simulink model "Copy_of_DFIG_Dynamic_Model"  (R2013a)
settings: Solver=ode45  StartTime=0.0  StopTime=30  RelTol=1e-3
values from neighbouring files (symbols this model uses):
  B = inv([ ... (first row only)    [WECSConstants.m]
  C = 14e-3    (= 0.014)    [WECSConstants.m]
  f = 60    [WECSConstants.m]
  Ki = 1    [WECSConstants.m]
  Kp = 3    [WECSConstants.m]
  Lg = Xg/wb    (= 0.000189434171015)    [WECSConstants.m]
  Lm = Xm/wb    (= 0.00249597832282)    [WECSConstants.m]
  Lr = Xr/wb    (= 0.00255883889524)    [WECSConstants.m]
  Ls = Xs/wb    (= 0.00255426721724)    [WECSConstants.m]
  P = 6    [WECSConstants.m]
  Pb = (2e6)/3    (= 666666.666667)    [WECSConstants.m]
  sigma = 1-(Lm*Lm)/(Ls*Lr)    (= 0.0468256531123)    [WECSConstants.m]
  Ts = 1    [WECSConstants.m]
  Vb = 690/(3^0.5)    (= 398.371685741)    [WECSConstants.m]
  VDC0 = 1200    [WECSConstants.m]
  wb = 2*pi*f    (= 376.991118431)    [WECSConstants.m]
  ws = wb    (= 376.991118431)    [WECSConstants.m]
  Xm_pu = 3.95279    [WECSConstants.m]
  Xr_pu = Xlr_pu+Xm_pu    (= 4.05234)    [WECSConstants.m]
  Z = [ ... (first row only)    [WECSConstants.m]
  Zb = Vb/Ib    (= 0.23805)    [WECSConstants.m]
undefined symbols (not defined in the file or in its folder): i, Kf, Tcomp
libraries: powerlib_extras x13, powerlib_meascontrol x2, simulink x1
settings Model: Creator=Sony  LastModifiedBy=Sony

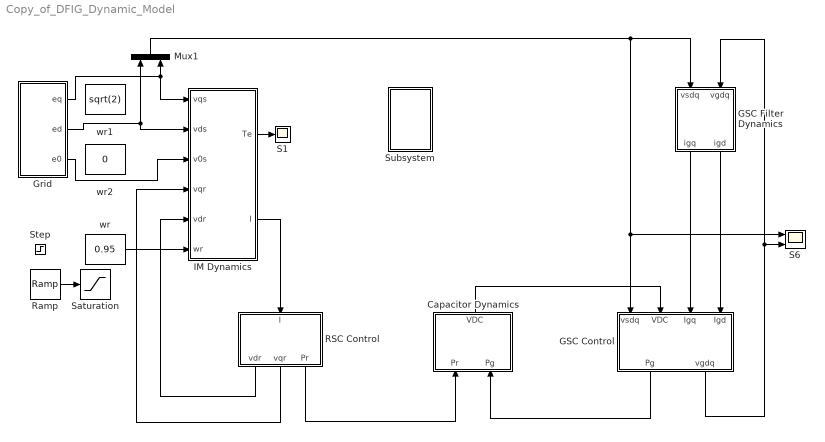
== system Copy_of_DFIG_Dynamic_Model ==
  Capacitor Dynamics : Subsystem
  GSC Control : Subsystem
  GSC Filter Dynamics : Subsystem
  Grid : Subsystem
  IM Dynamics : Subsystem
  Mux1 : Mux  Inputs=2
  RSC Control : Subsystem
  Ramp : simulink/Sources/Ramp  slope=1/5  start=1  X0=0
  S1 : Scope
      settings: SaveName=ScopeData14
  S6 : Scope  NumInputPorts=2
      settings: YMin=0~5.55112e-17  YMax=1.5~1.5  SaveName=ScopeData16
  Saturation : Saturate  UpperLimit=0.95
  Step : Step  Time=0  After=0.95  SampleTime=0
  Subsystem : Subsystem
  wr : Constant  Value=0.95
  wr1 : Constant  Value=sqrt(2)
  wr2 : Constant  Value=0
  wires:
  IM Dynamics/2(I) -> RSC Control/1(I)
  Grid/1(eq) -> IM Dynamics/1(vqs), Mux1/2
  RSC Control/1(vdr) -> IM Dynamics/5(vdr)
  RSC Control/2(vqr) -> IM Dynamics/4(vqr)
  RSC Control/3(Pr) -> Capacitor Dynamics/1(Pr)
  Capacitor Dynamics/1(VDC) -> GSC Control/2(VDC)
  GSC Control/1(Pg) -> Capacitor Dynamics/2(Pg)
  Mux1/1 -> GSC Filter Dynamics/1(vsdq), GSC Control/1(vsdq), S6/1
  GSC Control/2(vgdq) -> GSC Filter Dynamics/2(vgdq), S6/2
  GSC Filter Dynamics/1(igq) -> GSC Control/3(Igq)
  GSC Filter Dynamics/2(igd) -> GSC Control/4(Igd)
  IM Dynamics/1(Te) -> S1/1
  Ramp/1 -> Saturation/1
  wr/1 -> IM Dynamics/6(wr)
  Grid/2(ed) -> IM Dynamics/2(vds), Mux1/1
  Grid/3(e0) -> IM Dynamics/3(v0s)

== system Copy_of_DFIG_Dynamic_Model/Capacitor Dynamics ==
  Pr : Inport
  Pg : Inport  Port=2
  C1 : powerlib_extras/Discrete  Control Blocks/Discrete PI Controller  Kp=0  Ki=1/(C*VDC0)  Par_Limits=[1205 1195]  Init=1200  Ts=50e-6
  G : Gain  Gain=Pb
  G1 : Gain  Gain=1/Vb
  Mux : Mux  Inputs=3
  S2 : Scope
      settings: YMin=1190  YMax=1210  SaveName=ScopeData5
  S3 : Scope
      settings: YMin=-0.5  YMax=0.5  SaveName=ScopeData12
  Sum : Sum  Inputs=|--
  VDC : Outport
  wires:
  Sum/1 -> G/1
  Pr/1 -> Sum/1, Mux/2
  Pg/1 -> Sum/2, Mux/1
  C1/1 -> S2/1, G1/1
  G/1 -> C1/1
  G1/1 -> VDC/1
  [Qg] -> Mux/3
  Mux/1 -> S3/1

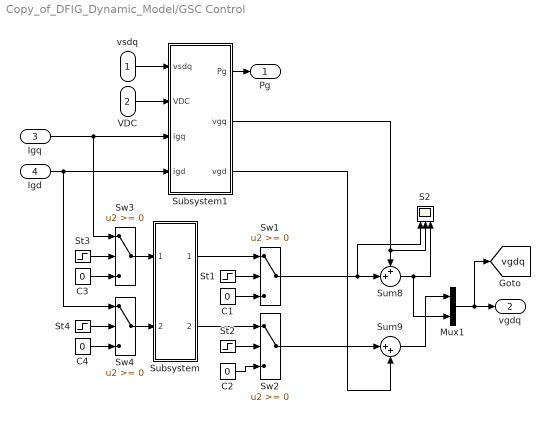
== system Copy_of_DFIG_Dynamic_Model/GSC Control ==
  vsdq : Inport
  VDC : Inport  Port=2
  Igq : Inport  Port=3
  Igd : Inport  Port=4
  C{1..4} (4 alike) : Constant  Value=0
  Mux1 : Mux  Inputs=2
  S2 : Scope  NumInputPorts=3
      settings: YMin=-10~0~1.4137  YMax=10~2~1.4147  SaveName=ScopeData53
  St{1..4} (4 alike) : Step  Time=Tcomp  Before=-1  SampleTime=0
  Subsystem : Subsystem
  Subsystem1 : Subsystem
  Sum8 : Sum  Inputs=++|
  Sum9 : Sum  Inputs=|++
  Sw1 : Switch  SampleTime=Ts
  Sw2 : Switch  SampleTime=Ts
  Sw3 : Switch
  Sw4 : Switch
  Pg : Outport
  vgdq : Outport  Port=2
  tag scope: vgdq=global
  wires:
  Mux1/1 -> [vgdq], vgdq/1
  vsdq/1 -> Subsystem1/1(vsdq)
  VDC/1 -> Subsystem1/2(VDC)
  Subsystem1/1(Pg) -> Pg/1
  Subsystem1/2(vgq) -> S2/2, Sum8/1
  Subsystem1/3(vgd) -> Sum9/2
  St1/1 -> Sw1/2
  C1/1 -> Sw1/3
  Subsystem/1(vgq) -> Sw1/1
  St2/1 -> Sw2/2
  C2/1 -> Sw2/3
  Subsystem/2(vgd) -> Sw2/1
  Sw1/1 -> S2/1, Sum8/2
  Sw2/1 -> Sum9/1
  Sum9/1 -> Mux1/1
  St3/1 -> Sw3/2
  C3/1 -> Sw3/3
  Igq/1 -> Subsystem1/3(igq), Sw3/1
  Sw3/1 -> Subsystem/1(igq)
  St4/1 -> Sw4/2
  C4/1 -> Sw4/3
  Igd/1 -> Sw4/1, Subsystem1/4(igd)
  Sw4/1 -> Subsystem/2(igd)
  Sum8/1 -> S2/3, Mux1/2

== system Copy_of_DFIG_Dynamic_Model/GSC Filter Dynamics ==
  vsdq : Inport
  vgdq : Inport  Port=2
  Add : Sum  Inputs=+-
  Add1 : Sum  Inputs=+-
  Demux : Demux  Outputs=2
  Demux1 : Demux  Outputs=2
  G : Gain
  G1 : Gain  Gain=-Zb/(wb*Lg)
  G2 : Gain  Gain=Zb/(wb*Lg)
  Mux2 : Mux  Inputs=2
  S1 : Scope  NumInputPorts=2
      settings: YMin=1.31236e+20~-5.13413e+16  YMax=1.4505e+20~-4.64517e+16  SaveName=ScopeData31
  S3 : Scope
      settings: YMin=-1  YMax=1  SaveName=ScopeData10
  igq : Outport
  igd : Outport  Port=2
  tag scope: igdq=global
  wires:
  vsdq/1 -> Demux1/1
  vgdq/1 -> Demux/1
  Demux1/2 -> Add/2
  Demux1/1 -> Add1/1
  Mux2/1 -> G/1
  G/1 -> [igdq], S3/1
  Demux/1 -> S1/1, Add1/2
  Demux/2 -> S1/2, Add/1
  G1/1 -> Mux2/2, igd/1
  G2/1 -> Mux2/1, igq/1
  Add/1 -> G1/1
  Add1/1 -> G2/1

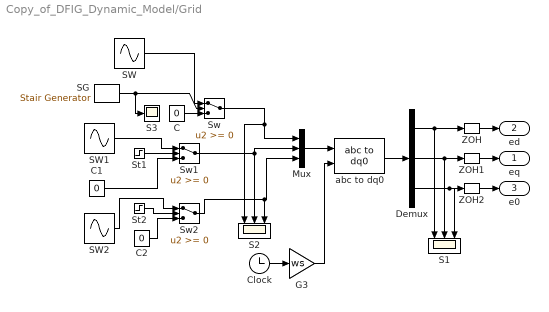
== system Copy_of_DFIG_Dynamic_Model/Grid ==
  C : Constant  Value=0
  C1 : Constant  Value=0
  C2 : Constant  Value=0
  Clock : Clock
  Demux : Demux  Outputs=3
  G3 : Gain  Gain=ws
  Mux : Mux  Inputs=3
  S1 : Scope  NumInputPorts=3
      settings: YMin=-1.5~-1.5~-1.5  YMax=1.5~1.5~1.5  SaveName=ScopeData19
  S2 : Scope  NumInputPorts=3
      settings: YMin=-1.5~-1.5~-1.5  YMax=1.5~1.5~1.5  SaveName=ScopeData21
  S3 : Scope
      settings: YMin=1  YMax=1  SaveName=ScopeData32
  SG : powerlib_meascontrol/Pulse & Signal Generators/Stair Generator  t=[0, 10, 15]  e=[1, -1, 1]  Ts=0
  SW : Sin  Amplitude=sqrt(2)  Frequency=ws  Phase=90*(pi/180)  SampleTime=0
  SW1 : Sin  Amplitude=sqrt(2)  Frequency=ws  Phase=-30*(pi/180)  SampleTime=0
  SW2 : Sin  Amplitude=sqrt(2)  Frequency=ws  Phase=-150*(pi/180)  SampleTime=0
  St1 : Step  Time=0  Before=-1  SampleTime=0
  St2 : Step  Time=0  Before=-1  SampleTime=0
  Sw : Switch
  Sw1 : Switch
  Sw2 : Switch
  ZOH : ZeroOrderHold
  ZOH1 : ZeroOrderHold
  ZOH2 : ZeroOrderHold
  abc to dq0 : powerlib_meascontrol/Transformations/abc to dq0  Alignment=90 degrees behind phase A axis
  eq : Outport
  ed : Outport  Port=2
  e0 : Outport  Port=3
  wires:
  Sw/1 -> S2/1, Mux/1
  Sw1/1 -> Mux/2, S2/2
  Mux/1 -> abc to dq0/1
  Clock/1 -> G3/1
  G3/1 -> abc to dq0/2
  Demux/1 -> ZOH/1, S1/1
  Demux/2 -> S1/2, ZOH1/1
  Demux/3 -> S1/3, ZOH2/1
  abc to dq0/1 -> Demux/1
  Sw2/1 -> S2/3, Mux/3
  SW/1 -> Sw/1
  C/1 -> Sw/3
  St1/1 -> Sw1/2
  C1/1 -> Sw1/3
  SW1/1 -> Sw1/1
  St2/1 -> Sw2/2
  C2/1 -> Sw2/3
  SW2/1 -> Sw2/1
  SG/1 -> S3/1, Sw/2
  ZOH/1 -> ed/1
  ZOH1/1 -> eq/1
  ZOH2/1 -> e0/1

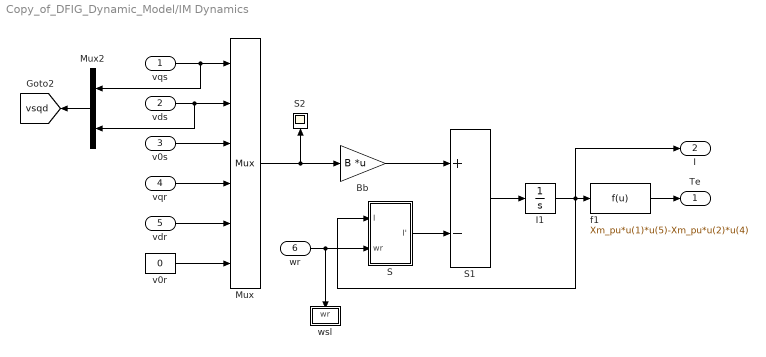
== system Copy_of_DFIG_Dynamic_Model/IM Dynamics ==
  vqs : Inport
  vds : Inport  Port=2
  v0s : Inport  Port=3
  vqr : Inport  Port=4
  vdr : Inport  Port=5
  wr : Inport  Port=6
  Bb : Gain  Gain=B  Multiplication=Matrix(K*u)
  I1 : Integrator  InitialCondition=[-0.5648; 0; 0; 0.578; 0.3585; 0]  UpperSaturationLimit=[2; 2; 2; 2; 2; 2]  LowerSaturationLimit=-[2; 2; 2; 2; 2; 2]
  Mux : Mux  Inputs=6
  Mux2 : Mux  Inputs=2
  S : Subsystem
  S1 : Sum  Inputs=+-
  S2 : Scope
      settings: YMin=950000  YMax=1.05e+06  SaveName=ScopeData8
  f1 : Fcn  Expr=Xm_pu*u(1)*u(5)-Xm_pu*u(2)*u(4)
  v0r : Constant  Value=0
  wsl : Subsystem
  Te : Outport
  I : Outport  Port=2
  tag scope: vsqd=global
  wires:
  S1/1 -> I1/1
  v0s/1 -> Mux/3
  f1/1 -> Te/1
  vdr/1 -> Mux/5
  Mux/1 -> Bb/1, S2/1
  vqr/1 -> Mux/4
  Bb/1 -> S1/1
  S/1(I') -> S1/2
  v0r/1 -> Mux/6
  I1/1 -> I/1, S/1(I), f1/1
  wr/1 -> S/2(wr), wsl/1(wr)
  vqs/1 -> Mux2/1, Mux/1
  vds/1 -> Mux2/2, Mux/2
  Mux2/1 -> [vsqd]

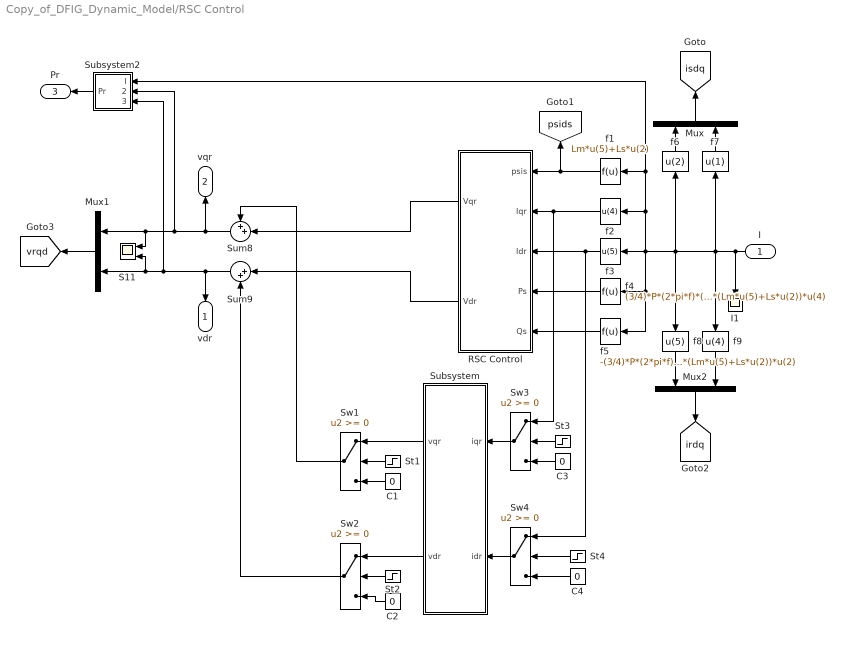
== system Copy_of_DFIG_Dynamic_Model/RSC Control ==
  I : Inport
  C{1..4} (4 alike) : Constant  Value=0
  I1 : Scope
      settings: YMin=-0.6  YMax=0.6
  Mux : Mux  Inputs=2
  Mux1 : Mux  Inputs=2
  Mux2 : Mux  Inputs=2
  RSC Control : Subsystem
  S11 : Scope  NumInputPorts=2
      settings: YMin=-1~-0.01  YMax=1~0.01  SaveName=ScopeData15
  St{1..4} (4 alike) : Step  Time=Tcomp  Before=-1  SampleTime=0
  Subsystem : Subsystem
  Subsystem2 : Subsystem
  Sum8 : Sum  Inputs=++|
  Sum9 : Sum  Inputs=|++
  Sw{1..4} (4 alike) : Switch
  f1 : Fcn  Expr=Lm*u(5)+Ls*u(2)
  f2 : Fcn  Expr=u(4)
  f3 : Fcn  Expr=u(5)
  f4 : Fcn  Expr=(3/4)*P*(2*pi*f)*(Lm/Ls)*(Lm*u(5)+Ls*u(2))*u(4)
  f5 : Fcn  Expr=-(3/4)*P*(2*pi*f)*(Lm*u(5)+Ls*u(2))*u(2)
  f6 : Fcn  Expr=u(2)
  f7 : Fcn  Expr=u(1)
  f8 : Fcn  Expr=u(5)
  f9 : Fcn  Expr=u(4)
  vdr : Outport
  vqr : Outport  Port=2
  Pr : Outport  Port=3
  tag scope: irdq=global, isdq=global, psids=global, vrqd=global
  wires:
  Subsystem2/1(Pr) -> Pr/1
  f1/1 -> RSC Control/1(psis), [psids]
  f4/1 -> RSC Control/4(Ps)
  f5/1 -> RSC Control/5(Qs)
  I/1 -> f5/1, f4/1, Subsystem2/1(I), f1/1, f2/1, f3/1, f8/1, f6/1, f9/1, f7/1, I1/1
  f6/1 -> Mux/1
  f7/1 -> Mux/2
  Mux/1 -> [isdq]
  RSC Control/2(Vdr) -> Sum9/1
  f8/1 -> Mux2/1
  f9/1 -> Mux2/2
  Mux2/1 -> [irdq]
  Subsystem/1(vqr) -> Sw1/1
  Subsystem/2(vdr) -> Sw2/1
  St1/1 -> Sw1/2
  C1/1 -> Sw1/3
  St2/1 -> Sw2/2
  C2/1 -> Sw2/3
  Sw1/1 -> Sum8/1
  Sw2/1 -> Sum9/2
  RSC Control/1(Vqr) -> Sum8/2
  Mux1/1 -> [vrqd]
  Sum8/1 -> Subsystem2/2(vqr), S11/1, Mux1/1, vqr/1
  Sum9/1 -> Subsystem2/3(vdr), S11/2, Mux1/2, vdr/1
  f2/1 -> Sw3/1, RSC Control/2(Iqr)
  St3/1 -> Sw3/2
  C3/1 -> Sw3/3
  Sw3/1 -> Subsystem/1(iqr)
  f3/1 -> Sw4/1, RSC Control/3(Idr)
  St4/1 -> Sw4/2
  C4/1 -> Sw4/3
  Sw4/1 -> Subsystem/2(idr)

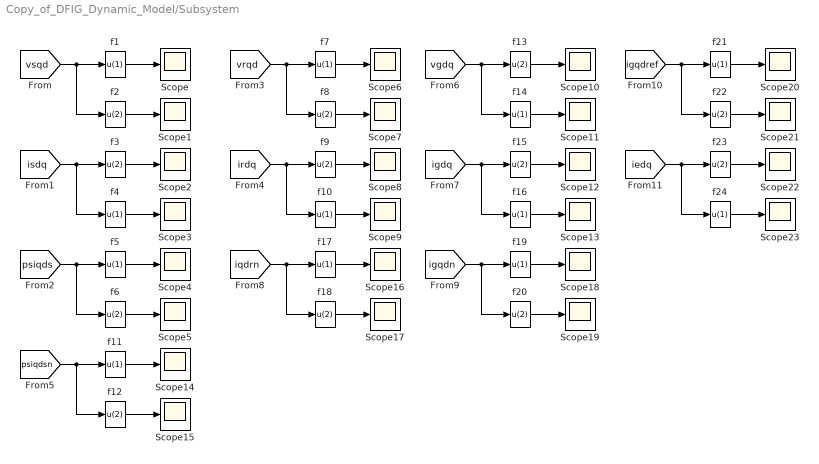
== system Copy_of_DFIG_Dynamic_Model/Subsystem ==
  Scope{,1..23} (24 alike) : Scope
      Scope settings: SaveName=ScopeData23
      Scope1 settings: SaveName=ScopeData26
      Scope10 settings: SaveName=ScopeData40
      Scope11 settings: YMin=0.00902765  YMax=0.00902835  SaveName=ScopeData41
      Scope12 settings: SaveName=ScopeData42
      Scope13 settings: SaveName=ScopeData43
      Scope14 settings: YMin=-0.0015  YMax=0.00125  SaveName=ScopeData38
      Scope15 settings: SaveName=ScopeData39
      Scope16 settings: YMin=-1  YMax=1  SaveName=ScopeData44
      Scope17 settings: YMin=-1  YMax=1  SaveName=ScopeData45
      Scope18 settings: YMin=-1e+25  YMax=1e+25  SaveName=ScopeData46
      Scope19 settings: YMin=-1e+25  YMax=1e+25  SaveName=ScopeData47
      Scope2 settings: SaveName=ScopeData27
      Scope20 settings: YMin=-11.2  YMax=10  SaveName=ScopeData48
      Scope21 settings: YMin=0.00902765  YMax=0.00902835  SaveName=ScopeData49
      Scope22 settings: YMin=-0.6  YMax=-0.275  SaveName=ScopeData50
      Scope23 settings: YMin=-1  YMax=1  SaveName=ScopeData51
      Scope3 settings: SaveName=ScopeData29
      Scope4 settings: SaveName=ScopeData30
      Scope5 settings: YMin=0.0008  YMax=0.001  SaveName=ScopeData33
      Scope6 settings: YMin=0.07000000000000001  YMax=0.08  SaveName=ScopeData34
      Scope7 settings: YMin=-1  YMax=1  SaveName=ScopeData35
      Scope8 settings: SaveName=ScopeData36
      Scope9 settings: SaveName=ScopeData37
  f{1,4..5,7,10..11,14,16..17,19,21,24} (12 alike) : Fcn  Expr=u(1)
  f{2..3,6,8..9,12..13,15,18,20,22..23} (12 alike) : Fcn  Expr=u(2)
  wires:
  [vsqd] -> f2/1, f1/1
  f1/1 -> Scope/1
  f2/1 -> Scope1/1
  [isdq] -> f4/1, f3/1
  f3/1 -> Scope2/1
  f4/1 -> Scope3/1
  [psiqds] -> f6/1, f5/1
  f5/1 -> Scope4/1
  f6/1 -> Scope5/1
  [vrqd] -> f8/1, f7/1
  f7/1 -> Scope6/1
  f8/1 -> Scope7/1
  [irdq] -> f10/1, f9/1
  f9/1 -> Scope8/1
  f10/1 -> Scope9/1
  [vgdq] -> f14/1, f13/1
  f13/1 -> Scope10/1
  f14/1 -> Scope11/1
  [igdq] -> f16/1, f15/1
  f15/1 -> Scope12/1
  f16/1 -> Scope13/1
  [psiqdsn] -> f12/1, f11/1
  f11/1 -> Scope14/1
  f12/1 -> Scope15/1
  [iqdrn] -> f18/1, f17/1
  f17/1 -> Scope16/1
  f18/1 -> Scope17/1
  [igqdn] -> f20/1, f19/1
  f19/1 -> Scope18/1
  f20/1 -> Scope19/1
  [igqdref] -> f22/1, f21/1
  f21/1 -> Scope20/1
  f22/1 -> Scope21/1
  [iedq] -> f24/1, f23/1
  f23/1 -> Scope22/1
  f24/1 -> Scope23/1

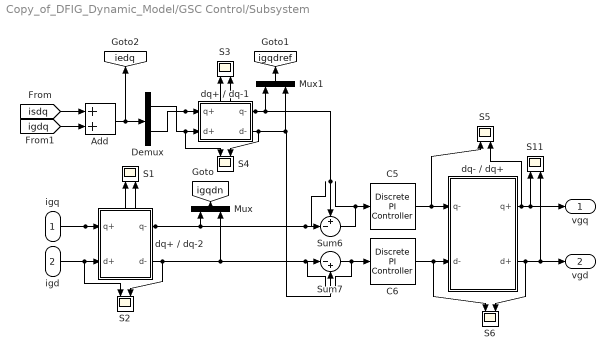
== system Copy_of_DFIG_Dynamic_Model/GSC Control/Subsystem ==
  igq : Inport
  igd : Inport  Port=2
  Add : Sum
  C5 : powerlib_extras/Discrete  Control Blocks/Discrete PI Controller  Kp=Kp  Ki=0  Par_Limits=[10e5 -10e5]  Init=0  Ts=50e-6
  C6 : powerlib_extras/Discrete  Control Blocks/Discrete PI Controller  Kp=Kp  Ki=0  Par_Limits=[10e5 -10e5]  Init=0  Ts=50e-6
  Demux : Demux  Outputs=2
  Mux : Mux  Inputs=2
  Mux1 : Mux  Inputs=2
  S{1..6,11} (7 alike) : Scope  NumInputPorts=2
      S1 settings: YMin=-1~-1  YMax=1~1  SaveName=ScopeData54
      S11 settings: YMin=-1.5~-1.5  YMax=1.5~1.5  SaveName=ScopeData28
      S2 settings: YMin=-1~-1  YMax=1~1  SaveName=ScopeData55
      S3 settings: YMin=-1~-1  YMax=1~1  SaveName=ScopeData56
      S4 settings: YMin=-1~-1  YMax=1~1  SaveName=ScopeData57
      S5 settings: YMin=-1~-1  YMax=1~1  SaveName=ScopeData58
      S6 settings: YMin=-1~-1  YMax=1~1  SaveName=ScopeData59
  Sum6 : Sum  Inputs=+-|
  Sum7 : Sum  Inputs=|-+
  dq+ / dq-1 : Subsystem
  dq+ / dq-2 : Subsystem
  dq- / dq+ : Subsystem
  vgq : Outport
  vgd : Outport  Port=2
  tag scope: iedq=global, igqdn=global, igqdref=global
  wires:
  Demux/1 -> S4/1, dq+ / dq-1/2(d+)
  dq+ / dq-1/2(d-) -> S4/2, Sum7/2, Mux1/2
  [isdq] -> Add/1
  dq- / dq+/1(q+) -> vgq/1, S11/1, S5/2
  dq- / dq+/2(d+) -> S6/2, S11/2, vgd/1
  [igdq] -> Add/2
  dq+ / dq-2/1(q-) -> Sum6/2, Mux/1, S1/2
  Add/1 -> Demux/1, [iedq]
  Sum7/1 -> C6/1
  Sum6/1 -> C5/1
  C5/1 -> S5/1, dq- / dq+/1(q-)
  dq+ / dq-2/2(d-) -> S2/2, Mux/2, Sum7/1
  C6/1 -> S6/1, dq- / dq+/2(d-)
  Demux/2 -> S3/1, dq+ / dq-1/1(q+)
  dq+ / dq-1/1(q-) -> S3/2, Sum6/1, Mux1/1
  igd/1 -> S2/1, dq+ / dq-2/2(d+)
  igq/1 -> S1/1, dq+ / dq-2/1(q+)
  Mux/1 -> [igqdn]
  Mux1/1 -> [igqdref]

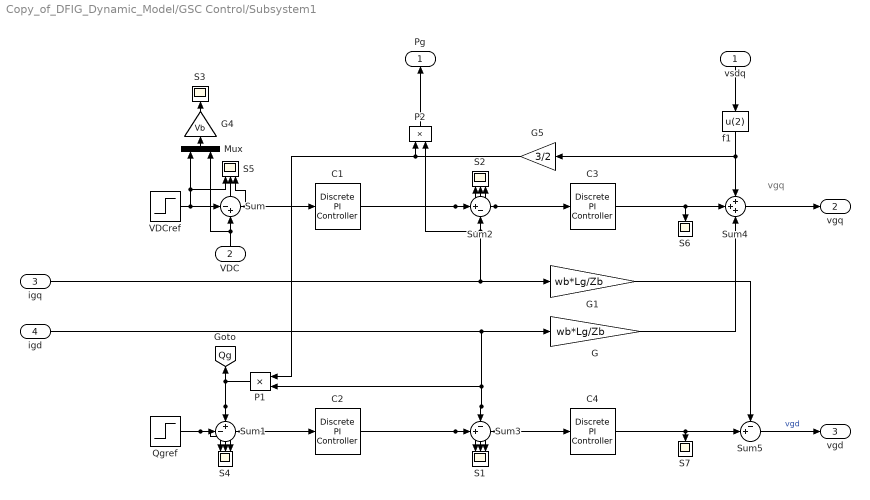
== system Copy_of_DFIG_Dynamic_Model/GSC Control/Subsystem1 ==
  note: vgq
  vsdq : Inport
  VDC : Inport  Port=2
  igq : Inport  Port=3
  igd : Inport  Port=4
  C1 : powerlib_extras/Discrete  Control Blocks/Discrete PI Controller  Kp=Kp  Ki=Ki  Par_Limits=[10e5 -10e5]  Init=0  Ts=Ts
  C2 : powerlib_extras/Discrete  Control Blocks/Discrete PI Controller  Kp=Kp  Ki=Ki  Par_Limits=[10e5 -10e5]  Init=0  Ts=Ts
  C3 : powerlib_extras/Discrete  Control Blocks/Discrete PI Controller  Kp=Kp  Ki=Ki  Par_Limits=[1e6 -1e6]  Init=0  Ts=Ts
  C4 : powerlib_extras/Discrete  Control Blocks/Discrete PI Controller  Kp=Kp  Ki=Ki  Par_Limits=[1e6 -1e6]  Init=0  Ts=Ts
  G : Gain  Gain=wb*Lg/Zb
  G1 : Gain  Gain=wb*Lg/Zb
  G4 : Gain  Gain=Vb
  G5 : Gain  Gain=3/2
  Mux : Mux  Inputs=2
  P1 : Product
  P2 : Product
  Qgref : Step  Time=0  After=0  SampleTime=0
  S{1..2,4..5} (4 alike) : Scope  NumInputPorts=3
      S1 settings: YMin=-1.05e+06~-4.11888e+22~3.7266e+22  YMax=-950000~-3.7266e+22~4.11888e+22  SaveName=ScopeData6
      S2 settings: YMin=0.0357706~-5.87597e+28~5.31635e+28  YMax=0.039536~-5.31635e+28~5.87597e+28  SaveName=ScopeData2
      S4 settings: YMin=-0.25~-0.25~-0.25  YMax=0.25~0.25~0.25  SaveName=ScopeData9
      S5 settings: YMin=2.99~2.99~-0.02  YMax=3.04~3.04~0.02  SaveName=ScopeData11
  S3 : Scope
      settings: YMin=1190  YMax=1210  SaveName=ScopeData22
  S6 : Scope
      settings: TimeRange=0.1  YMin=-1  YMax=1  SaveName=ScopeData24
  S7 : Scope
      settings: TimeRange=50  YMin=-1  YMax=1  SaveName=ScopeData25
  Sum : Sum  Inputs=|-+
  Sum1 : Sum  Inputs=+-|
  Sum2 : Sum  Inputs=|+-
  Sum3 : Sum  Inputs=-+|
  Sum4 : Sum  Inputs=+++
  Sum5 : Sum  Inputs=-+|
  VDCref : Step  Time=0  Before=1200/Vb  After=1200/Vb  SampleTime=0
  f1 : Fcn  Expr=u(2)
  Pg : Outport
  vgq : Outport  Port=2
  vgd : Outport  Port=3
  tag scope: Qg=global
  wires:
  P1/1 -> S4/2, Sum1/1, [Qg]
  Sum3/1 -> C4/1, S1/3
  Sum2/1 -> C3/1, S2/3
  C2/1 -> S1/1, Sum3/2
  VDCref/1 -> S5/1, Mux/1, Sum/1
  VDC/1 -> Mux/2, S5/2, Sum/2
  G5/1 -> P1/1, P2/1
  Sum1/1 -> C2/1, S4/3
  C1/1 -> Sum2/1, S2/1
  C4/1 -> Sum5/2, S7/1
  Qgref/1 -> S4/1, Sum1/2
  G4/1 -> S3/1
  C3/1 -> S6/1, Sum4/2
  G1/1 -> Sum5/1
  vsdq/1 -> f1/1
  Sum5/1 -> vgd/1  "vgd"
  G/1 -> Sum4/3
  Mux/1 -> G4/1
  Sum/1 -> C1/1, S5/3
  f1/1 -> Sum4/1, G5/1
  P2/1 -> Pg/1
  Sum4/1 -> vgq/1
  igq/1 -> S2/2, P2/2, Sum2/2, G1/1
  igd/1 -> Sum3/1, S1/2, P1/2, G/1

== system Copy_of_DFIG_Dynamic_Model/IM Dynamics/S ==
  I : Inport
  wr : Inport  Port=2
  G1 : Gain  Gain=Z  Multiplication=Matrix(K*u)
  G2 : Gain  Gain=B  Multiplication=Matrix(K*u)
  G3 : Gain  Gain=[0 0 0 0 0 0;0 0 0 0 0 0;0 0 0 0 0 0;0 -Xm_pu 0 0 -Xr_pu 0;Xm_pu 0 0 Xr_pu 0 0;0 0 0 0 0 0]
  Matrix Sum : Sum
  P : Product  Multiplication=Matrix(*)
  I' : Outport
  wires:
  G2/1 -> I'/1
  P/1 -> Matrix Sum/2
  Matrix Sum/1 -> G2/1
  G3/1 -> P/1
  G1/1 -> Matrix Sum/1
  I/1 -> P/2, G1/1
  wr/1 -> G3/1

== system Copy_of_DFIG_Dynamic_Model/IM Dynamics/wsl ==
  wr : Inport
  Add1 : Sum  Inputs=+-
  Gain : Gain  Gain=1/wb
  Scope1 : Scope
      settings: YMin=0.9025  YMax=0.9975  SaveName=ScopeData13
  Scope2 : Scope
      settings: YMin=0.0475  YMax=0.0525  SaveName=ScopeData18
  wr1 : Constant
  tag scope: wsl=global
  wires:
  wr/1 -> Scope1/1, Add1/2
  Add1/1 -> Scope2/1, [wsl]
  [we] -> Gain/1
  wr1/1 -> Add1/1

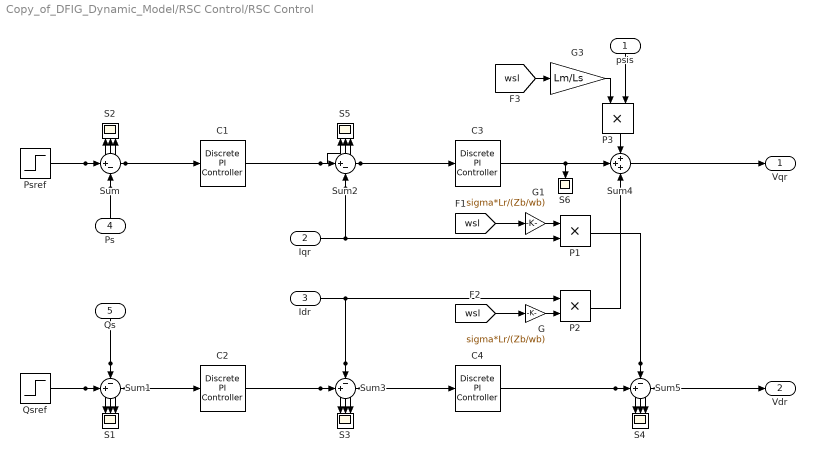
== system Copy_of_DFIG_Dynamic_Model/RSC Control/RSC Control ==
  psis : Inport
  Iqr : Inport  Port=2
  Idr : Inport  Port=3
  Ps : Inport  Port=4
  Qs : Inport  Port=5
  C1 : powerlib_extras/Discrete  Control Blocks/Discrete PI Controller  Kp=Kp  Ki=Ki  Par_Limits=[10e5 -10e5]  Init=0  Ts=50e-6
  C2 : powerlib_extras/Discrete  Control Blocks/Discrete PI Controller  Kp=Kp  Ki=Ki  Par_Limits=[10e5 -10e5]  Init=0  Ts=50e-6
  C3 : powerlib_extras/Discrete  Control Blocks/Discrete PI Controller  Kp=Kp  Ki=Ki  Par_Limits=[10e5 -10e5]  Init=0.0724  Ts=50e-6
  C4 : powerlib_extras/Discrete  Control Blocks/Discrete PI Controller  Kp=Kp  Ki=Ki  Par_Limits=[10e5 -10e5]  Init=1.968e-3  Ts=50e-6
  G : Gain  Gain=sigma*Lr/(Zb/wb)
  G1 : Gain  Gain=sigma*Lr/(Zb/wb)
  G3 : Gain  Gain=Lm/Ls
  P1 : Product
  P2 : Product
  P3 : Product
  Psref : Step  Time=0  Before=0.95*0.95*0.95  After=0.95*0.95*0.95  SampleTime=0
  Qsref : Step  Time=0  After=0  SampleTime=0
  S{1..5} (5 alike) : Scope  NumInputPorts=3
      S1 settings: YMin=-1~-1~-1  YMax=1~1~1  SaveName=ScopeData4
      S2 settings: YMin=0.814506~0.6~-0.3  YMax=0.900244~1.15~0.25  SaveName=ScopeData3
      S3 settings: YMin=0.358236~0.358234~7.5e-07  YMax=0.358241~0.358239~3e-06  SaveName=ScopeData7
      S4 settings: YMin=0.00196795~0.00548418~-0.00351623  YMax=0.00196805~0.00548419~-0.00351613  SaveName=ScopeData17
      S5 settings: YMin=0.5772~0.5776~-0.0005  YMax=0.5789~0.57845~0.0005  SaveName=ScopeData20
  S6 : Scope
      settings: YMin=0.0723587  YMax=0.0723622
  Sum : Sum  Inputs=|+-
  Sum1 : Sum  Inputs=-+|
  Sum2 : Sum  Inputs=|+-
  Sum3 : Sum  Inputs=-+|
  Sum4 : Sum  Inputs=+++
  Sum5 : Sum  Inputs=-+|
  Vqr : Outport
  Vdr : Outport  Port=2
  wires:
  Psref/1 -> S2/1, Sum/1
  Ps/1 -> S2/2, Sum/2
  Qsref/1 -> S1/1, Sum1/2
  Qs/1 -> S1/2, Sum1/1
  Sum/1 -> C1/1, S2/3
  P3/1 -> Sum4/1
  Sum3/1 -> C4/1, S3/3
  G1/1 -> P1/1
  Sum2/1 -> C3/1, S5/3
  Sum1/1 -> C2/1, S1/3
  C4/1 -> S4/1, Sum5/2
  Iqr/1 -> S5/2, Sum2/2, P1/2
  Idr/1 -> S3/2, Sum3/1, P2/1
  C2/1 -> S3/1, Sum3/2
  C3/1 -> S6/1, Sum4/2
  Sum4/1 -> Vqr/1
  Sum5/1 -> Vdr/1, S4/3
  [wsl] -> G1/1
  [wsl] -> G/1
  P1/1 -> S4/2, Sum5/1
  P2/1 -> Sum4/3
  G3/1 -> P3/1
  psis/1 -> P3/2
  [wsl] -> G3/1
  C1/1 -> S5/1, Sum2/1
  G/1 -> P2/2

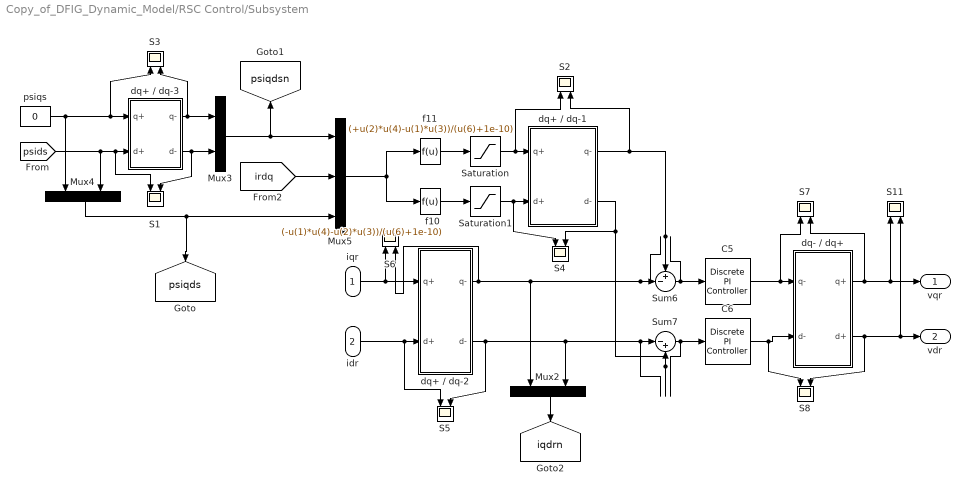
== system Copy_of_DFIG_Dynamic_Model/RSC Control/Subsystem ==
  iqr : Inport
  idr : Inport  Port=2
  C5 : powerlib_extras/Discrete  Control Blocks/Discrete PI Controller  Kp=Kp  Ki=Ki  Par_Limits=[10e5 -10e5]  Init=0  Ts=50e-6
  C6 : powerlib_extras/Discrete  Control Blocks/Discrete PI Controller  Kp=Kp  Ki=Ki  Par_Limits=[10e5 -10e5]  Init=0  Ts=50e-6
  Mux2 : Mux  Inputs=2
  Mux3 : Mux  Inputs=2
  Mux4 : Mux  Inputs=2
  Mux5 : Mux  Inputs=3
  S{1..8,11} (9 alike) : Scope  NumInputPorts=2
      S1 settings: YMin=-1~-1  YMax=1~1  SaveName=ScopeData61
      S11 settings: YMin=-0.5~-0.5  YMax=1.5~1.5  SaveName=ScopeData28
      S2 settings: YMin=-1~-1  YMax=1~1  SaveName=ScopeData62
      S3 settings: YMin=-1~-1  YMax=1~1  SaveName=ScopeData60
      S4 settings: YMin=-1~-1  YMax=1~1  SaveName=ScopeData63
      S5 settings: YMin=-1~-0.0009  YMax=1~0.0011  SaveName=ScopeData64
      S6 settings: YMin=-1~-1  YMax=1~1  SaveName=ScopeData65
      S7 settings: YMin=-1~-1  YMax=1~1  SaveName=ScopeData66
      S8 settings: YMin=-1~-1  YMax=1~1  SaveName=ScopeData67
  Saturation : Saturate  UpperLimit=1e6  LowerLimit=-1e6
  Saturation1 : Saturate  UpperLimit=1e6  LowerLimit=-1e6
  Sum6 : Sum  Inputs=+-|
  Sum7 : Sum  Inputs=|-+
  dq+ / dq-1 : Subsystem
  dq+ / dq-2 : Subsystem
  dq+ / dq-3 : Subsystem
  dq- / dq+ : Subsystem
  f10 : Fcn  Expr=(-u(1)*u(4)-u(2)*u(3))/(u(6)+1e-10)
  f11 : Fcn  Expr=(+u(2)*u(4)-u(1)*u(3))/(u(6)+1e-10)
  psiqs : Constant  Value=0
  vqr : Outport
  vdr : Outport  Port=2
  tag scope: iqdrn=global, psiqds=global, psiqdsn=global
  wires:
  dq+ / dq-1/2(d-) -> S4/2, Sum7/2
  dq- / dq+/1(q+) -> S7/2, vqr/1, S11/1
  dq- / dq+/2(d+) -> S8/2, vdr/1, S11/2
  dq+ / dq-2/1(q-) -> Sum6/2, Mux2/1, S6/2
  Sum7/1 -> C6/1
  Sum6/1 -> C5/1
  C5/1 -> S7/1, dq- / dq+/1(q-)
  dq+ / dq-2/2(d-) -> S5/2, Sum7/1, Mux2/2
  C6/1 -> S8/1, dq- / dq+/2(d-)
  dq+ / dq-1/1(q-) -> S2/2, Sum6/1
  idr/1 -> S5/1, dq+ / dq-2/2(d+)
  psiqs/1 -> S3/1, dq+ / dq-3/1(q+), Mux4/1
  [psids] -> S1/1, dq+ / dq-3/2(d+), Mux4/2
  dq+ / dq-3/1(q-) -> S3/2, Mux3/1
  dq+ / dq-3/2(d-) -> S1/2, Mux3/2
  Mux3/1 -> [psiqdsn], Mux5/1
  [irdq] -> Mux5/2
  Mux5/1 -> f11/1, f10/1
  Mux4/1 -> [psiqds], Mux5/3
  f11/1 -> Saturation/1
  f10/1 -> Saturation1/1
  Mux2/1 -> [iqdrn]
  Saturation/1 -> S2/1, dq+ / dq-1/1(q+)
  Saturation1/1 -> S4/1, dq+ / dq-1/2(d+)
  iqr/1 -> S6/1, dq+ / dq-2/1(q+)

== system Copy_of_DFIG_Dynamic_Model/RSC Control/Subsystem2 ==
  I : Inport
  vqr : Inport  Port=2
  vdr : Inport  Port=3
  A : Sum
  G : Gain  Gain=3/2
  P1 : Product
  P2 : Product
  f6 : Fcn  Expr=u(4)
  f7 : Fcn  Expr=u(5)
  Pr : Outport
  wires:
  P2/1 -> A/2
  G/1 -> Pr/1
  f6/1 -> P1/1
  I/1 -> f7/1, f6/1
  P1/1 -> A/1
  f7/1 -> P2/1
  vdr/1 -> P2/2
  vqr/1 -> P1/2
  A/1 -> G/1

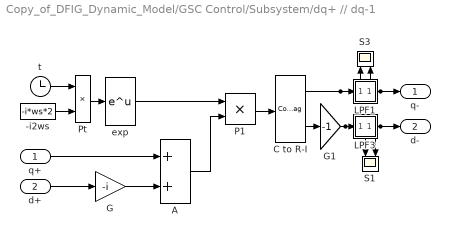
== system Copy_of_DFIG_Dynamic_Model/GSC Control/Subsystem/dq+ // dq-1 ==
  q+ : Inport
  d+ : Inport  Port=2
  -i2ws : Constant  Value=-i*ws*2
  A : Sum
  C to R-I : ComplexToRealImag
  G : Gain  Gain=-i
  G1 : Gain  Gain=-1
  LPF1 : Subsystem
  LPF3 : Subsystem
  P1 : Product
  Pt : Product
  S1 : Scope  NumInputPorts=2
      settings: YMin=-1~-1  YMax=1~1  SaveName=ScopeData69
  S3 : Scope  NumInputPorts=2
      settings: YMin=-1~-1  YMax=1~1  SaveName=ScopeData68
  exp : Math  OutputSignalType=complex  SaturateOnIntegerOverflow=on
  t : Clock
  q- : Outport
  d- : Outport  Port=2
  wires:
  C to R-I/2 -> G1/1
  t/1 -> Pt/1
  -i2ws/1 -> Pt/2
  Pt/1 -> exp/1
  exp/1 -> P1/1
  G/1 -> A/2
  q+/1 -> A/1
  A/1 -> P1/2
  P1/1 -> C to R-I/1
  d+/1 -> G/1
  C to R-I/1 -> LPF1/1(I), S3/1
  G1/1 -> LPF3/1(I), S1/1
  LPF1/1(O) -> q-/1, S3/2
  LPF3/1(O) -> d-/1, S1/2

== system Copy_of_DFIG_Dynamic_Model/GSC Control/Subsystem/dq+ // dq-2 ==
  q+ : Inport
  d+ : Inport  Port=2
  -i2ws : Constant  Value=-i*ws*2
  A : Sum
  C to R-I : ComplexToRealImag
  G : Gain  Gain=-i
  G1 : Gain  Gain=-1
  LPF1 : Subsystem
  LPF3 : Subsystem
  P1 : Product
  Pt : Product
  S11 : Scope  NumInputPorts=2
      settings: YMin=-0.1~-0.01  YMax=0.1~0.01  SaveName=ScopeData52
  S3 : Scope  NumInputPorts=2
      settings: YMin=-1~-0.01  YMax=1~0.01  SaveName=ScopeData70
  exp : Math  OutputSignalType=complex  SaturateOnIntegerOverflow=on
  t : Clock
  q- : Outport
  d- : Outport  Port=2
  wires:
  C to R-I/2 -> G1/1
  t/1 -> Pt/1
  -i2ws/1 -> Pt/2
  Pt/1 -> exp/1
  exp/1 -> P1/1
  G/1 -> A/2
  q+/1 -> A/1
  A/1 -> P1/2
  P1/1 -> C to R-I/1
  d+/1 -> G/1
  C to R-I/1 -> LPF1/1(I), S11/1
  G1/1 -> LPF3/1(I), S3/1
  LPF1/1(O) -> S11/2, q-/1
  LPF3/1(O) -> d-/1, S3/2

== system Copy_of_DFIG_Dynamic_Model/GSC Control/Subsystem/dq- // dq+ ==
  q- : Inport
  d- : Inport  Port=2
  Add : Sum
  Complex to Real-Imag : ComplexToRealImag
  Gain : Gain  Gain=-i
  Gain1 : Gain  Gain=-1
  LPF2 : Subsystem
  LPF4 : Subsystem
  Product : Product
  Product1 : Product
  S1 : Scope  NumInputPorts=2
      settings: YMin=-1~-1  YMax=1~1  SaveName=ScopeData72
  S3 : Scope  NumInputPorts=2
      settings: YMin=-1~-1  YMax=1~1  SaveName=ScopeData71
  exp : Math  SaturateOnIntegerOverflow=on
  i2ws : Constant  Value=i*ws*2
  t : Clock
  q+ : Outport
  d+ : Outport  Port=2
  wires:
  Complex to Real-Imag/2 -> Gain1/1
  t/1 -> Product/1
  i2ws/1 -> Product/2
  Product/1 -> exp/1
  exp/1 -> Product1/1
  d-/1 -> Gain/1
  Gain/1 -> Add/2
  q-/1 -> Add/1
  Add/1 -> Product1/2
  Product1/1 -> Complex to Real-Imag/1
  Complex to Real-Imag/1 -> LPF4/1(I), S3/1
  Gain1/1 -> LPF2/1(I), S1/1
  LPF4/1(O) -> S3/2, q+/1
  LPF2/1(O) -> S1/2, d+/1

== system Copy_of_DFIG_Dynamic_Model/RSC Control/Subsystem/dq+ // dq-1 ==
  q+ : Inport
  d+ : Inport  Port=2
  -i2ws : Constant  Value=-i*ws*2
  A : Sum
  C to R-I : ComplexToRealImag
  G : Gain  Gain=-i
  G1 : Gain  Gain=-1
  LPF1 : Subsystem
  LPF3 : Subsystem
  P1 : Product
  Pt : Product
  S1 : Scope  NumInputPorts=2
      settings: YMin=-1~-1  YMax=1~1  SaveName=ScopeData74
  S3 : Scope  NumInputPorts=2
      settings: YMin=-1~-1  YMax=1~1  SaveName=ScopeData73
  exp : Math  OutputSignalType=complex  SaturateOnIntegerOverflow=on
  t : Clock
  q- : Outport
  d- : Outport  Port=2
  wires:
  C to R-I/2 -> G1/1
  t/1 -> Pt/1
  -i2ws/1 -> Pt/2
  Pt/1 -> exp/1
  exp/1 -> P1/1
  G/1 -> A/2
  q+/1 -> A/1
  A/1 -> P1/2
  P1/1 -> C to R-I/1
  d+/1 -> G/1
  C to R-I/1 -> LPF1/1(I), S3/1
  G1/1 -> LPF3/1(I), S1/1
  LPF1/1(O) -> q-/1, S3/2
  LPF3/1(O) -> d-/1, S1/2

== system Copy_of_DFIG_Dynamic_Model/RSC Control/Subsystem/dq+ // dq-2 ==
  q+ : Inport
  d+ : Inport  Port=2
  -i2ws : Constant  Value=-i*ws*2
  A : Sum
  C to R-I : ComplexToRealImag
  G : Gain  Gain=-i
  G1 : Gain  Gain=-1
  LPF1 : Subsystem
  LPF3 : Subsystem
  P1 : Product
  Pt : Product
  S1 : Scope  NumInputPorts=2
      settings: YMin=-1~-1  YMax=1~1  SaveName=ScopeData76
  S3 : Scope  NumInputPorts=2
      settings: YMin=-1~-1  YMax=1~1  SaveName=ScopeData75
  exp : Math  OutputSignalType=complex  SaturateOnIntegerOverflow=on
  t : Clock
  q- : Outport
  d- : Outport  Port=2
  wires:
  C to R-I/2 -> G1/1
  t/1 -> Pt/1
  -i2ws/1 -> Pt/2
  Pt/1 -> exp/1
  exp/1 -> P1/1
  G/1 -> A/2
  q+/1 -> A/1
  A/1 -> P1/2
  P1/1 -> C to R-I/1
  d+/1 -> G/1
  C to R-I/1 -> LPF1/1(I), S3/1
  G1/1 -> LPF3/1(I), S1/1
  LPF1/1(O) -> S3/2, q-/1
  LPF3/1(O) -> S1/2, d-/1

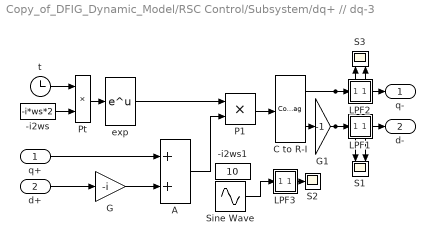
== system Copy_of_DFIG_Dynamic_Model/RSC Control/Subsystem/dq+ // dq-3 ==
  q+ : Inport
  d+ : Inport  Port=2
  -i2ws : Constant  Value=-i*ws*2
  -i2ws1 : Constant  Value=10
  A : Sum
  C to R-I : ComplexToRealImag
  G : Gain  Gain=-i
  G1 : Gain  Gain=-1
  LPF1 : Subsystem
  LPF2 : Subsystem
  LPF3 : Subsystem
  P1 : Product
  Pt : Product
  S1 : Scope  NumInputPorts=2
      settings: YMin=-1~-1  YMax=1~1  SaveName=ScopeData78
  S2 : Scope
      settings: YMin=-4  YMax=6  SaveName=ScopeData81
  S3 : Scope  NumInputPorts=2
      settings: YMin=-1~-1  YMax=1~1  SaveName=ScopeData77
  Sine Wave : Sin  Amplitude=10  Bias=1  Frequency=2*pi*30  SampleTime=0
  exp : Math  OutputSignalType=complex  SaturateOnIntegerOverflow=on
  t : Clock
  q- : Outport
  d- : Outport  Port=2
  wires:
  C to R-I/2 -> G1/1
  t/1 -> Pt/1
  -i2ws/1 -> Pt/2
  Pt/1 -> exp/1
  exp/1 -> P1/1
  G/1 -> A/2
  q+/1 -> A/1
  A/1 -> P1/2
  P1/1 -> C to R-I/1
  d+/1 -> G/1
  C to R-I/1 -> LPF2/1(I), S3/1
  G1/1 -> LPF1/1(I), S1/1
  LPF2/1(O) -> S3/2, q-/1
  LPF1/1(O) -> S1/2, d-/1
  Sine Wave/1 -> LPF3/1(I)
  LPF3/1(O) -> S2/1

== system Copy_of_DFIG_Dynamic_Model/RSC Control/Subsystem/dq- // dq+ ==
  q- : Inport
  d- : Inport  Port=2
  Add : Sum
  Complex to Real-Imag : ComplexToRealImag
  Gain : Gain  Gain=-i
  Gain1 : Gain  Gain=-1
  LPF1 : Subsystem
  LPF3 : Subsystem
  Product : Product
  Product1 : Product
  S1 : Scope  NumInputPorts=2
      settings: YMin=-1~-1  YMax=1~1  SaveName=ScopeData80
  S3 : Scope  NumInputPorts=2
      settings: YMin=-1~-1  YMax=1~1  SaveName=ScopeData79
  exp : Math  SaturateOnIntegerOverflow=on
  i2ws : Constant  Value=i*ws*2
  t : Clock
  q+ : Outport
  d+ : Outport  Port=2
  wires:
  Complex to Real-Imag/2 -> Gain1/1
  t/1 -> Product/1
  i2ws/1 -> Product/2
  Product/1 -> exp/1
  exp/1 -> Product1/1
  d-/1 -> Gain/1
  Gain/1 -> Add/2
  q-/1 -> Add/1
  Add/1 -> Product1/2
  Product1/1 -> Complex to Real-Imag/1
  Complex to Real-Imag/1 -> LPF1/1(I), S3/1
  LPF1/1(O) -> q+/1, S3/2
  Gain1/1 -> LPF3/1(I), S1/1
  LPF3/1(O) -> S1/2, d+/1

== system Copy_of_DFIG_Dynamic_Model/GSC Control/Subsystem/dq+ // dq-1/LPF1 ==
  I : Inport
  Gain : Gain  Gain=Kf
  Gain1 : Gain  Gain=Kf
  Integrator : Integrator
  Sum : Sum  Inputs=|+-
  O : Outport
  wires:
  Sum/1 -> Integrator/1
  Integrator/1 -> O/1, Gain/1
  I/1 -> Gain1/1
  Gain/1 -> Sum/2
  Gain1/1 -> Sum/1

== system Copy_of_DFIG_Dynamic_Model/GSC Control/Subsystem/dq+ // dq-1/LPF3 ==
  I : Inport
  Gain : Gain  Gain=Kf
  Gain1 : Gain  Gain=Kf
  Integrator : Integrator
  Sum : Sum  Inputs=|+-
  O : Outport
  wires:
  Sum/1 -> Integrator/1
  Integrator/1 -> O/1, Gain/1
  I/1 -> Gain1/1
  Gain/1 -> Sum/2
  Gain1/1 -> Sum/1

== system Copy_of_DFIG_Dynamic_Model/GSC Control/Subsystem/dq+ // dq-2/LPF1 ==
  I : Inport
  Gain : Gain  Gain=Kf
  Gain1 : Gain  Gain=Kf
  Integrator : Integrator
  Sum : Sum  Inputs=|+-
  O : Outport
  wires:
  Sum/1 -> Integrator/1
  Integrator/1 -> O/1, Gain/1
  I/1 -> Gain1/1
  Gain/1 -> Sum/2
  Gain1/1 -> Sum/1

== system Copy_of_DFIG_Dynamic_Model/GSC Control/Subsystem/dq+ // dq-2/LPF3 ==
  I : Inport
  Gain : Gain  Gain=Kf
  Gain1 : Gain  Gain=Kf
  Integrator : Integrator
  Sum : Sum  Inputs=|+-
  O : Outport
  wires:
  Sum/1 -> Integrator/1
  Integrator/1 -> O/1, Gain/1
  I/1 -> Gain1/1
  Gain/1 -> Sum/2
  Gain1/1 -> Sum/1

== system Copy_of_DFIG_Dynamic_Model/GSC Control/Subsystem/dq- // dq+/LPF2 ==
  I : Inport
  Gain : Gain  Gain=Kf
  Gain1 : Gain  Gain=Kf
  Integrator : Integrator
  Sum : Sum  Inputs=|+-
  O : Outport
  wires:
  Sum/1 -> Integrator/1
  Integrator/1 -> O/1, Gain/1
  I/1 -> Gain1/1
  Gain/1 -> Sum/2
  Gain1/1 -> Sum/1

== system Copy_of_DFIG_Dynamic_Model/GSC Control/Subsystem/dq- // dq+/LPF4 ==
  I : Inport
  Gain : Gain  Gain=Kf
  Gain1 : Gain  Gain=Kf
  Integrator : Integrator
  Sum : Sum  Inputs=|+-
  O : Outport
  wires:
  Sum/1 -> Integrator/1
  Integrator/1 -> O/1, Gain/1
  I/1 -> Gain1/1
  Gain/1 -> Sum/2
  Gain1/1 -> Sum/1

== system Copy_of_DFIG_Dynamic_Model/RSC Control/Subsystem/dq+ // dq-1/LPF1 ==
  I : Inport
  Gain : Gain  Gain=Kf
  Gain1 : Gain  Gain=Kf
  Integrator : Integrator
  Sum : Sum  Inputs=|+-
  O : Outport
  wires:
  Sum/1 -> Integrator/1
  Integrator/1 -> O/1, Gain/1
  I/1 -> Gain1/1
  Gain/1 -> Sum/2
  Gain1/1 -> Sum/1

== system Copy_of_DFIG_Dynamic_Model/RSC Control/Subsystem/dq+ // dq-1/LPF3 ==
  I : Inport
  Gain : Gain  Gain=Kf
  Gain1 : Gain  Gain=Kf
  Integrator : Integrator
  Sum : Sum  Inputs=|+-
  O : Outport
  wires:
  Sum/1 -> Integrator/1
  Integrator/1 -> O/1, Gain/1
  I/1 -> Gain1/1
  Gain/1 -> Sum/2
  Gain1/1 -> Sum/1

== system Copy_of_DFIG_Dynamic_Model/RSC Control/Subsystem/dq+ // dq-2/LPF1 ==
  I : Inport
  Gain : Gain  Gain=Kf
  Gain1 : Gain  Gain=Kf
  Integrator : Integrator
  Sum : Sum  Inputs=|+-
  O : Outport
  wires:
  Sum/1 -> Integrator/1
  Integrator/1 -> O/1, Gain/1
  I/1 -> Gain1/1
  Gain/1 -> Sum/2
  Gain1/1 -> Sum/1

== system Copy_of_DFIG_Dynamic_Model/RSC Control/Subsystem/dq+ // dq-2/LPF3 ==
  I : Inport
  Gain : Gain  Gain=Kf
  Gain1 : Gain  Gain=Kf
  Integrator : Integrator
  Sum : Sum  Inputs=|+-
  O : Outport
  wires:
  Sum/1 -> Integrator/1
  Integrator/1 -> O/1, Gain/1
  I/1 -> Gain1/1
  Gain/1 -> Sum/2
  Gain1/1 -> Sum/1

== system Copy_of_DFIG_Dynamic_Model/RSC Control/Subsystem/dq+ // dq-3/LPF1 ==
  I : Inport
  Gain : Gain  Gain=Kf
  Gain1 : Gain  Gain=Kf
  Integrator : Integrator
  Sum : Sum  Inputs=|+-
  O : Outport
  wires:
  Sum/1 -> Integrator/1
  Integrator/1 -> O/1, Gain/1
  I/1 -> Gain1/1
  Gain/1 -> Sum/2
  Gain1/1 -> Sum/1

== system Copy_of_DFIG_Dynamic_Model/RSC Control/Subsystem/dq+ // dq-3/LPF2 ==
  I : Inport
  Gain : Gain  Gain=Kf
  Gain1 : Gain  Gain=Kf
  Integrator : Integrator
  Sum : Sum  Inputs=|+-
  O : Outport
  wires:
  Sum/1 -> Integrator/1
  Integrator/1 -> O/1, Gain/1
  I/1 -> Gain1/1
  Gain/1 -> Sum/2
  Gain1/1 -> Sum/1

== system Copy_of_DFIG_Dynamic_Model/RSC Control/Subsystem/dq+ // dq-3/LPF3 ==
  I : Inport
  Gain : Gain  Gain=Kf
  Gain1 : Gain  Gain=Kf
  Integrator : Integrator
  Sum : Sum  Inputs=|+-
  O : Outport
  wires:
  Sum/1 -> Integrator/1
  Integrator/1 -> O/1, Gain/1
  I/1 -> Gain1/1
  Gain/1 -> Sum/2
  Gain1/1 -> Sum/1

== system Copy_of_DFIG_Dynamic_Model/RSC Control/Subsystem/dq- // dq+/LPF1 ==
  I : Inport
  Gain : Gain  Gain=Kf
  Gain1 : Gain  Gain=Kf
  Integrator : Integrator
  Sum : Sum  Inputs=|+-
  O : Outport
  wires:
  Sum/1 -> Integrator/1
  Integrator/1 -> O/1, Gain/1
  I/1 -> Gain1/1
  Gain/1 -> Sum/2
  Gain1/1 -> Sum/1

== system Copy_of_DFIG_Dynamic_Model/RSC Control/Subsystem/dq- // dq+/LPF3 ==
  I : Inport
  Gain : Gain  Gain=Kf
  Gain1 : Gain  Gain=Kf
  Integrator : Integrator
  Sum : Sum  Inputs=|+-
  O : Outport
  wires:
  Sum/1 -> Integrator/1
  Integrator/1 -> O/1, Gain/1
  I/1 -> Gain1/1
  Gain/1 -> Sum/2
  Gain1/1 -> Sum/1
